simulink model "Offline_SCGAnalysis_AverageCycleCalculator"  (R2019a)
settings: Solver=FixedStepDiscrete  StartTime=0.0  StopTime=param_sim_time  FixedStep=1/fs  MaxStep=1/fs  RelTol=1e-3
undefined symbols (not defined in the file): analyses
settings Model: PacingRate=100  Creator=rcord  LastModifiedBy=rcord
settings SolverCC: ZeroCrossControl=DisableAll
settings DataIOCC: ExternalInput=[t, signals.scg.preprocessing_x, signals.scg.preprocessing_y, signals.scg.preprocessing_z]  LoadExternalInput=on  SignalLogging=off  DSMLogging=off  SaveTime=off  ReturnWorkspaceOutputs=off  TimeSaveName=t_preprocessing  OutputSaveName=out_preprocessing  LoggingIntervals=[-inf,inf]

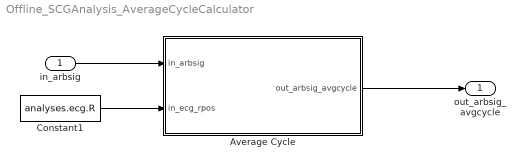
== system Offline_SCGAnalysis_AverageCycleCalculator ==
  in_arbsig : Inport
  Average Cycle : Subsystem
  Constant1 : Constant  Value=analyses.ecg.R
  out_arbsig_avgcycle : Outport
  wires:
  in_arbsig/1 -> Average Cycle/1(in_arbsig)
  Constant1/1 -> Average Cycle/2(in_ecg_rpos)
  Average Cycle/1(out_arbsig_avgcycle) -> out_arbsig_avgcycle/1

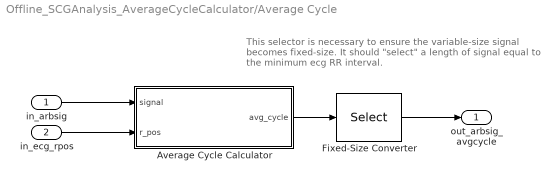
== system Offline_SCGAnalysis_AverageCycleCalculator/Average Cycle ==
  note: This selector is necessary to ensure the variable-size signal
      | becomes fixed-size. It should "select" a length of signal equal
      | to the minimum ecg RR interval.
  in_arbsig : Inport
  in_ecg_rpos : Inport  Port=2
  Average Cycle Calculator : MATLAB Function  TreatAsAtomicUnit=on
  Fixed-Size Converter : Selector  NumberOfDimensions=2  IndexOptions=Index vector (dialog),Index vector (dialog)  Indices=[1:min(analyses.ecg.RR)],1  OutputSizes=1,1
  out_arbsig_avgcycle : Outport
  wires:
  Average Cycle Calculator/1(avg_cycle) -> Fixed-Size Converter/1
  Fixed-Size Converter/1 -> out_arbsig_avgcycle/1
  in_ecg_rpos/1 -> Average Cycle Calculator/2(r_pos)
  in_arbsig/1 -> Average Cycle Calculator/1(signal)

== matlab function Offline_SCGAnalysis_AverageCycleCalculator/Average Cycle/Average Cycle Calculator ==
  data: signal input; r_pos input; avg_cycle output size=[min(analyses.ecg.RR) 1]
function avg_cycle  = avg_cycle_calculator(signal, r_pos)
% Simulink function to return the average cycle of an arbitraty signal input.

% INPUTS:
% r_pos = index positions of the R peaks of the ecg.
% signal = arbitrary input signal.

% OUTPUT:
% avg_cycle = averaged cycle of arbitrary input signal.


% Calculating number of cycles to be considered in averaging
rr_min = min(diff(r_pos)); % Shortest cycle length - all the cycles will but cut down to this length.

if length(signal) > r_pos(end) + rr_min
    considered_cycles = length(r_pos);
else
    considered_cycles = length(r_pos) - 1;
end

signal_cycles = zeros(rr_min,considered_cycles);

fig_average_cycle = figure;

% Isolating and plotting each cycle
for i = 1:considered_cycles
    figure(fig_average_cycle);
    signal_cycles(:,i) = signal(r_pos(i):r_pos(i) + rr_min - 1,1);
    plot(signal_cycles(:,i),'b'); hold on
end

% Calculating average cycle
avg_cycle = mean(signal_cycles,2);

% Plotting the average cycle
plot(avg_cycle,'k','LineWidth',2); title('Average Cycle'); xlabel('Time (msec)'); ylabel('Acceleration (mg)'); box off;
title('3D Modulus')
end
